simulink library "AR_Drone_Sensors"  (R2016a)
settings: Solver=ode45  StartTime=0.0  StopTime=10.0  RelTol=1e-3
settings Model: Creator=sannem  LastModifiedBy=sannem
settings DataIOCC: LimitDataPoints=on
settings DebuggingCC: AllowSymbolicDim=off

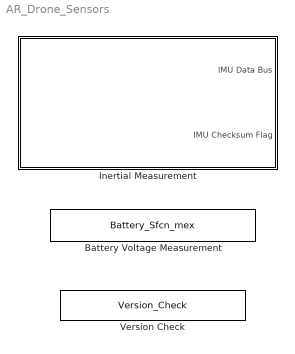
== system AR_Drone_Sensors ==
  Battery Voltage Measurement : S-Function  FunctionName=Battery_Sfcn_mex  Parameters=SampleTime  SFunctionDeploymentMode=off  EnableBusSupport=off  mask(Read Battery Voltage){SFunctionSpec=void BatteryMeasure_step(single y1[1]), SampleTime=-1}
      mask prompts: SampleTime "Sample time (-1 for inherited):"
      mask help:
      | Using I2C, this block reads Battery Voltage from ADCIN0 on the AR Drone 2.0's main board.
      |
      | From reading raw ADC values, one can observe a a linear response
      | 9.0V = 662	9.5V = 698	10.0V = 737
      | 10.5V=774	11.0V = 811	11.5V = 848
      | 12.0V=886	12.5V = 923
      | This leads to the 0.13595166 magic number for conversion to decivolt.
      |
      | To convert to regular voltage (V) units, divide the output of this block by 10.
      mask Display: fprintf('Battery Voltage Measurement [dV]');
  Inertial Measurement : Subsystem  mask{Ts=1/200}
      mask help: The ARM Cortex A9 SOC connects to this navigation board (PIC16 Microcontroller) over a serial cable connection. This has already been connected by default. The PIC microcontroller reads in sensor data which will handle the ADC readings. One thing to note is that the IMU board controlled by the PIC microcontroller operates at 200 Hz. If this block is set to a sample rate below that, it has been noted that packets will occasionally drop, especially in External Mode. To that end, it is better to sample this block at a higher sample rate above 200 Hz such that we do not get fragmented data packets. If the sample rate is too low the data might become fragmented and will consider that a 'lost' packet
      mask Help:
      | The ARM Cortex A9 SOC connects to this navigation board (PIC16 Microcontroller) over a serial cable connection. This has already been connected by default. The PIC microcontroller reads in sensor data which will handle the ADC readings. One thing to note is that the IMU board controlled by the PIC microcontroller operates at 200 Hz. If this block is set to a sample rate below that, it has been noted that packets will occasionally drop, especially in External Mode. To that end, it is better to sample this block at a higher sample rate above 200 Hz such that we do not get fragmented data packets. If the sample rate is too low the data might become fragmented and will consider that a 'lost' packet
      | 
      | The complete navigation 'struct' or bus signal looks like this:
      | 
      |  typedef struct  __attribute__ ((packed)){
      |         uint16_t taille;
      |         uint16_t nu_trame;
      | 
      |         uint16_t ax;
      |         uint16_t ay;
      |         uint16_t az;
      | 
      |         int16_t vx;
      |         int16_t vy;
      |         int16_t vz;
      |         uint16_t temperature_acc;
      |         uint16_t temperature_gyro;
      | 
      |         uint16_t ultrasound;
      | 
      |         uint16_t us_debut_echo;
      |         uint16_t us_fin_echo;
      |         uint16_t us_association_echo;
      |         uint16_t us_distance_echo;
      | 
      |         uint16_t us_curve_time;
      |         uint16_t us_curve_value;
      |         uint16_t us_curve_ref;
      | 
      |         uint16_t nb_echo;
      | 
      |         uint32_t sum_echo; //unsigned long
      |         int16_t gradient;
      | 
      |         uint16_t flag_echo_ini;
      | 
      |         int32_t pressure;
      |         uint16_t temperature_pressure;
      | 
      |         int16_t my;
      |         int16_t mx;
      |         int16_t mz;
      | 
      |         uint16_t chksum;
      | 
      |     }IMU_Packets;
      mask DialogControl DescGroupVar Prompt: Inertial Measurement Unit Block
      mask DialogControl DescTextVar Prompt: This block will output a bus signal containing data directly from the Inertial Measurement Unit board. The four major measurements include 3-axis sensors readings of the Rate Gyro, Accelerometer, Magnetometer. A scalar ultrasound altimeter reading provides relative distance to the ground. The IMU data bus includes many other readings include barometer, temperature sensing and a wide range of other sensor readings
      mask DialogControl Control3 Prompt: The ARM Cortex A9 SOC connects to this navigation board (PIC16 Microcontroller) over a serial cable connection. This has already been connected by default. The PIC microcontroller reads in sensor data which will handle the ADC readings. One thing to note is that the IMU board controlled by the PIC microcontroller operates at 200 Hz. If this block is set to a sample rate below that, it has been noted that packets will occasionally drop, especially in External Mode. To that end, it is better to sample this block at a higher sample rate above 200 Hz such that we do not get fragmented data packets. If the sample rate is too low the data might become fragmented and will consider that a 'lost' packet
      mask DialogControl Control5 Prompt: A checksum flag output has been provided to indicate when the checksum fails, which can be attributed to packet loss.
      mask DialogControl Control2 Prompt: Sample Time
      mask DialogControl Load_Bus_Obj Prompt: Load Navigation Bus Object From Library
      mask DialogControl Load_Bus_Obj Callback:
      | LibPath = which('AR_Drone_2_Library');
      | MagicValue = regexp(LibPath,'AR_Drone_2_Library.slx');
      | 
      | load([LibPath(1:(MagicValue-1)) 'Save_IMU_struct.mat'])
      | clear LibPath;
      | clear MagicValue;
      mask Display:
      | fprintf('Rate Gyro \n Accelerometer \n Magnetometer \n Ultrasound Altimeter')
      | port_label('output',1,'IMU Data Bus')
      | port_label('output',2,'IMU Checksum Flag')
  Version Check : S-Function  FunctionName=Version_Check  SFunctionDeploymentMode=off  EnableBusSupport=off  mask(Legacy Function){SFunctionSpec=void versionCheckStep(uint8 y1[1]), ShowSpec=on}
      mask prompts: ShowSpec "Display function specification"
      mask help: This block checks the version of the AR Drone Firmware using the update/version.txt file located on the AR Drone. If the AR Drone is running a supported version of the firmware (2.4.8) the block ouputs 1, else it outputs 0.
      mask Help: <p>This block was generated automatically by the Legacy Code Tool. For detailed help on this tool, call<a href="matlab:legacy_code('help')"> legacy_code('help')</a>.</p>
      mask Callback ShowSpec:
      | if strcmp(get_param(gcbh, 'ShowSpec'), 'on')
      |   set_param(gcbh, 'MaskDisplay', sprintf('fprintf(''%s'');', get_param(gcbh, 'SFunctionSpec')));
      | else
      |   set_param(gcbh, 'MaskDisplay', sprintf('fprintf(''%s'');', get_param(gcbh, 'FunctionName')));
      | end
      mask Display: fprintf('Version Check');

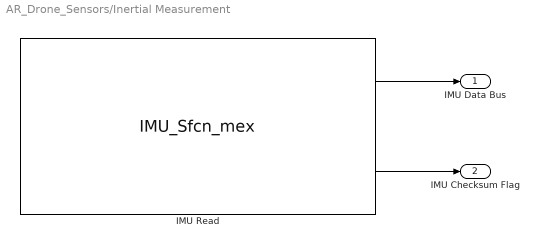
== system AR_Drone_Sensors/Inertial Measurement ==
  IMU Read : S-Function  FunctionName=IMU_Sfcn_mex  Parameters=SampleTime  SFunctionDeploymentMode=off  EnableBusSupport=off  mask(Legacy Function){SFunctionSpec=void MDL_IMU_step(IMU_Packets y1[1], int32 y2[1]), SampleTime=Ts, ShowSpec=on}
      mask prompts: SampleTime "Sample time (-1 for inherited):"; ShowSpec "Display function specification"
      mask help:
      | This block allows you to call the legacy functions specified by the following Legacy Code Tool definition:
      | def.SFunctionName = 'IMU_Sfcn_mex';
      | def.InitializeConditionsFcnSpec = 'void MDL_IMU_start()';
      | def.OutputFcnSpec = 'void MDL_IMU_step(IMU_Packets y1[1], int32 y2[1])';
      | def.TerminateFcnSpec = 'void MDL_IMU_term()';
      | def.SourceFiles = {'IMU_Navdata_Wrapper.c'};
      | def.SampleTime = 'parameterized';
      | def.Options.useTlcWithAccel = false;
      mask Help: <p>This block was generated automatically by the Legacy Code Tool. For detailed help on this tool, call<a href="matlab:legacy_code('help')"> legacy_code('help')</a>.</p>
      mask Callback ShowSpec:
      | if strcmp(get_param(gcbh, 'ShowSpec'), 'on')
      |   set_param(gcbh, 'MaskDisplay', sprintf('fprintf(''%s'');', get_param(gcbh, 'SFunctionSpec')));
      | else
      |   set_param(gcbh, 'MaskDisplay', sprintf('fprintf(''%s'');', get_param(gcbh, 'FunctionName')));
      | end
      mask Display: fprintf('void MDL_IMU_step(IMU_Packets y1[1], int32 y2[1])');
  IMU Data Bus : Outport
  IMU Checksum Flag : Outport  Port=2
  wires:
  IMU Read/1 -> IMU Data Bus/1
  IMU Read/2 -> IMU Checksum Flag/1
